simulink model "NEXTWAYPOINT"  (R2022b)
settings: Solver=VariableStepAuto  StartTime=0.0  StopTime=10.0  RelTol=1e-3
settings Model: Creator=lucaerviati  LastModifiedBy=lucaerviati
settings DataIOCC: SaveOutput=off  SaveTime=off
settings GRTTargetCC: CombineOutputUpdateFcns=off  MatFileLogging=off

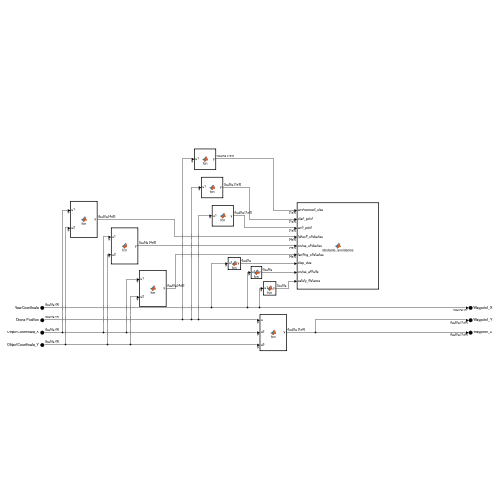
[thumbnail: Simulink's stored preview of the top-level diagram]
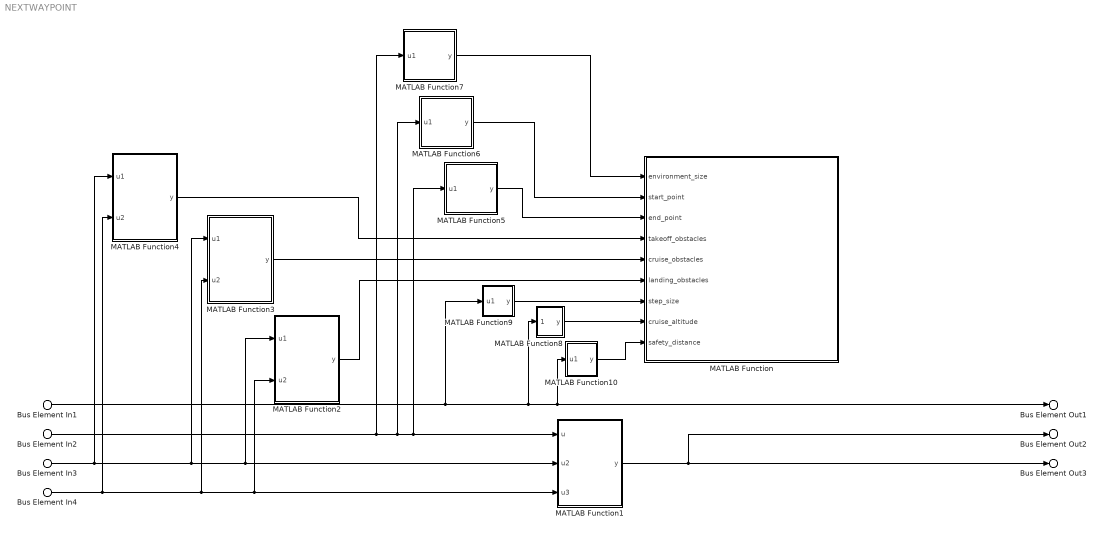
== system NEXTWAYPOINT ==
  Bus Element In1 : Inport  PortName=NewCoordinate
  Bus Element In2 : Inport  Port=2  PortName=Drone Position
  Bus Element In3 : Inport  Port=3  PortName=ObjectCoordinate_X
  Bus Element In4 : Inport  Port=4  PortName=ObjectCoordinate_Y
  MATLAB Function : MATLAB Function  TreatAsAtomicUnit=on
  MATLAB Function1 : MATLAB Function  TreatAsAtomicUnit=on
  MATLAB Function10 : MATLAB Function  TreatAsAtomicUnit=on
  MATLAB Function2 : MATLAB Function  TreatAsAtomicUnit=on
  MATLAB Function3 : MATLAB Function  TreatAsAtomicUnit=on
  MATLAB Function4 : MATLAB Function  TreatAsAtomicUnit=on
  MATLAB Function5 : MATLAB Function  TreatAsAtomicUnit=on
  MATLAB Function6 : MATLAB Function  TreatAsAtomicUnit=on
  MATLAB Function7 : MATLAB Function  TreatAsAtomicUnit=on
  MATLAB Function8 : MATLAB Function  TreatAsAtomicUnit=on
  MATLAB Function9 : MATLAB Function  TreatAsAtomicUnit=on
  Bus Element Out1 : Outport  PortName=Waypoint_X
  Bus Element Out2 : Outport  Port=2  PortName=Waypoint_Y
  Bus Element Out3 : Outport  Port=3  PortName=Waypoint_Z
  wires:
  MATLAB Function6/1(y) -> MATLAB Function/2(start_point)
  MATLAB Function5/1(y) -> MATLAB Function/3(end_point)
  MATLAB Function7/1(y) -> MATLAB Function/1(environment_size)
  MATLAB Function10/1(y) -> MATLAB Function/9(safety_distance)
  MATLAB Function8/1(y) -> MATLAB Function/8(cruise_altitude)
  MATLAB Function4/1(y) -> MATLAB Function/4(takeoff_obstacles)
  Bus Element In1/1 -> MATLAB Function8/1(u1), MATLAB Function10/1(u1), Bus Element Out1/1, MATLAB Function9/1(u1)
  Bus Element In2/1 -> MATLAB Function7/1(u1), MATLAB Function6/1(u1), MATLAB Function5/1(u1), MATLAB Function1/1(u)
  MATLAB Function1/1(y) -> Bus Element Out3/1, Bus Element Out2/1
  Bus Element In3/1 -> MATLAB Function4/1(u1), MATLAB Function3/1(u1), MATLAB Function1/2(u2), MATLAB Function2/1(u1)
  Bus Element In4/1 -> MATLAB Function4/2(u2), MATLAB Function3/2(u2), MATLAB Function1/3(u3), MATLAB Function2/2(u2)
  MATLAB Function2/1(y) -> MATLAB Function/6(landing_obstacles)
  MATLAB Function3/1(y) -> MATLAB Function/5(cruise_obstacles)
  MATLAB Function9/1(y) -> MATLAB Function/7(step_size)

== matlab function NEXTWAYPOINT/MATLAB Function10 ==
  data: u1 input; y output
function y = fcn(u1)

u = 6;
y=u;
end

== matlab function NEXTWAYPOINT/MATLAB Function1 ==
  data: u input; y output; u2 input; u3 input
function y = fcn(u,u2,u3)

u = 1;
if u>0
    y = [1,2,30,4,1,1,12,3,4];
else
    y = [0,2,30,4,1,1,12,3,4];
end

== matlab function NEXTWAYPOINT/MATLAB Function ==
  data: environment_size input; start_point input; end_point input; takeoff_obstacles input; cruise_obstacles input; landing_obstacles input; step_size input; cruise_altitude input; safety_distance input
function obstacle_avoidance(environment_size, start_point, end_point, takeoff_obstacles, cruise_obstacles, landing_obstacles, step_size, cruise_altitude, safety_distance)
    % Define points for different flight phases
    takeoff_end_point = [start_point(1), start_point(2), cruise_altitude];
    cruise_start_point = takeoff_end_point;
    cruise_end_point = [end_point(1), end_point(2), cruise_altitude];
    landing_start_point = cruise_end_point;

    % Create figure for real-time plotting
    hFig = figure;
    hold on;
    xlabel('X'); ylabel('Y'); zlabel('Z');
    grid on;
    title('Drone Flight Simulation');
    axis([0 environment_size(1) 0 environment_size(2) 0 environment_size(3)]);
    view(3);

    % Plot obstacles
    plot3(takeoff_obstacles(:,1), takeoff_obstacles(:,2), takeoff_obstacles(:,3), 'rx', 'MarkerSize', 10, 'LineWidth', 2);
    plot3(cruise_obstacles(:,1), cruise_obstacles(:,2), cruise_obstacles(:,3), 'rx', 'MarkerSize', 10, 'LineWidth', 2);
    plot3(landing_obstacles(:,1), landing_obstacles(:,2), landing_obstacles(:,3), 'rx', 'MarkerSize', 10, 'LineWidth', 2);

    % Function to check if a point is within safety distance of any obstacles
    function is_near = is_near_obstacle(point, obstacles)
        distances = sqrt(sum((obstacles - point).^2, 2));
        is_near = any(distances < safety_distance);
    end

    % Function to avoid obstacles by adjusting the point
    function adjusted_point = avoid_obstacles(point, obstacles)
        if is_near_obstacle(point, obstacles)
            % Calculate direction away from obstacles
            away_direction = sum((point - obstacles) ./ sqrt(sum((point - obstacles).^2, 2)), 1);
            away_direction = away_direction / norm(away_direction);
            % Adjust point along the away direction
            adjusted_point = point + away_direction * step_size;
        else
            adjusted_point = point;
        end
    end

    % Takeoff path with obstacle avoidance
    takeoff_path = [linspace(start_point(1), takeoff_end_point(1), 30)', ...
                    linspace(start_point(2), takeoff_end_point(2), 30)', ...
                    linspace(start_point(3), takeoff_end_point(3), 30)'];
    for i = 1:size(takeoff_path, 1)
        point = takeoff_path(i, :);
        while is_near_obstacle(point, takeoff_obstacles)
            point = avoid_obstacles(point, takeoff_obstacles);
        end
        plot3(point(1), point(2), point(3), 'b.', 'MarkerSize', 10); % Takeoff path in blue
        drawnow; % Update the plot in real time
        pause(0.1); % Pause to simulate real-time plotting
    end

    % Cruise path with obstacle avoidance
    cruise_path = [linspace(cruise_start_point(1), cruise_end_point(1), 100)', ...
                   linspace(cruise_start_point(2), cruise_end_point(2), 100)', ...
                   linspace(cruise_start_point(3), cruise_end_point(3), 100)'];
    for i = 1:size(cruise_path, 1)
        point = cruise_path(i, :);
        while is_near_obstacle(point, cruise_obstacles)
            point = avoid_obstacles(point, cruise_obstacles);
        end
        plot3(point(1), point(2), point(3), 'k.', 'MarkerSize', 10); % Cruise path in black
        drawnow; % Update the plot in real time
        pause(0.1); % Pause to simulate real-time plotting
        
        % Check if drone has landed
        if norm(point - end_point) < safety_distance
            break; % Exit the loop if drone has landed
        end
    end

    % Landing path with obstacle avoidance
    landing_path = [linspace(landing_start_point(1), end_point(1), 30)', ...
                    linspace(landing_start_point(2), end_point(2), 30)', ...
                    linspace(landing_start_point(3), end_point(3), 30)'];
    for i = 1:size(landing_path, 1)
        point = landing_path(i, :);
        while is_near_obstacle(point, landing_obstacles)
            point = avoid_obstacles(point, landing_obstacles);
        end
        plot3(point(1), point(2), point(3), 'g.', 'MarkerSize', 10); % Landing path in green
        drawnow; % Update the plot in real time
        pause(0.1); % Pause to simulate real-time plotting
        
        % Check if drone has landed
        if norm(point - end_point) < safety_distance
            break; % Exit the loop if drone has landed
        end
    end

    hold off;
end

== matlab function NEXTWAYPOINT/MATLAB Function2 ==
  data: u1 input; y output; u2 input
function y = fcn(u1, u2)

u = [85, 85, 5;80, 80, 10;75, 75, 0;90, 70, 0];
y=u;
end

== matlab function NEXTWAYPOINT/MATLAB Function3 ==
  data: u1 input; y output; u2 input
function y = fcn(u1, u2)

u = [ 50, 50, 50;60, 60, 60;55, 55, 45;65, 45, 55];
y=u;
end

== matlab function NEXTWAYPOINT/MATLAB Function4 ==
  data: u1 input; y output; u2 input
function y = fcn(u1, u2)

u = [15, 15, 15;20, 20, 20;25, 25, 10;30, 15, 20];
y=u;
end

== matlab function NEXTWAYPOINT/MATLAB Function5 ==
  data: u1 input; y output
function y = fcn(u1)

u = [90, 90, 0];
y=u;
end

== matlab function NEXTWAYPOINT/MATLAB Function6 ==
  data: u1 input; y output
function y = fcn(u1)

u = [10, 10, 10];
y=u;
end

== matlab function NEXTWAYPOINT/MATLAB Function7 ==
  data: u1 input; y output
function y = fcn(u1)

u = [100, 100, 100];
y=u;
end

== matlab function NEXTWAYPOINT/MATLAB Function8 ==
  data: u1 input; y output
function y = fcn(u1)

u = 50;
y=u;
end

== matlab function NEXTWAYPOINT/MATLAB Function9 ==
  data: u1 input; y output
function y = fcn(u1)

u = 1;
y=u;
end
